simulink model "Demo_DSRC_BSM_Message_cs"  (Simulink 8.7)
settings: Solver=ode5  SolverMode=SingleTasking  StartTime=0.0  StopTime=10  FixedStep=1/20  RelTol=1e-3
PreLoadFcn:
  | check_NUTS_defined;
  | 
  | assignin('base',['model_closed_' bdroot],false);
InitFcn:
  | PreScanExperimentInitFcn(bdroot)
StopFcn:
  | PreScanExperimentStopFcn(bdroot)
undefined symbols (not defined in the file): spare_1, spare_10, spare_11, spare_12, spare_13, spare_14, spare_15, spare_16, spare_17, spare_18, spare_19, spare_2, spare_3, spare_4, spare_5, spare_6, spare_7, spare_8, spare_9
libraries: PreScanSimulinkLibrary x12, PreScanUsefulBlocks x4, simulink x2
(part 2 of 3)

== system Demo_DSRC_BSM_Message_cs/BMW_Z3_1/Trajectories ==
  Traj2State1 : Subsystem  Tag=Traj2State  mask(PreScan Demux Block:){}
      settings: DeleteFcn=PreScanBlockDeleteFcn;
  Trajectory_1 : Subsystem  Tag=Trajectory  mask(PreScan Source Block: Trajectory){FileName='Trajectory_1.mat', TimeStep=1/20}
      mask prompts: TimeStep "Time Step [s]"
      mask help:
      | The Trajectory block contains the trajectories defined in the PreScan Experiment Editor. The output of the trajectory block is the (vehicle) State.
      |
      | For more information, please click Help.
      mask init:
      | [direc,name]=fileparts(get_param(bdroot, 'FileName'));
      | load([direc,'/Trajectories/',FileName])
      | trajectory=trajectory';
      | 
      | traj.time=trajectory(:,1);%[];
      | traj.signals.values=trajectory(:,2:19);
      | traj.dimensions=18;
      | traj.label='';
      | 
      | SampleTime=traj.time(2)-traj.time(1);
      settings: DeleteFcn=PreScanBlockDeleteFcn;
      mask Help: eval('openHelp(312)')
      mask Display: fprintf(FileName)
  Trajectory_1_Offset : Constant  Tag=TrajectoryOffset  Value="[0  0  0  0  0  0]"
  State : Outport  Tag=TrajOutport
  wires:
  Trajectory_1/1(trajectory) -> Traj2State1/1(Traj Org)
  Trajectory_1_Offset/1 -> Traj2State1/2(Offset)
  Traj2State1/1(state) -> State/1

== system Demo_DSRC_BSM_Message_cs/Citroen_C3_1/DSRC Transmitter ==
  Data : Inport
  Enable : EnablePort  PropagateVarSize=During execution
  DSRC_T_BusAssignment : BusAssignment  Tag=BusDSRCT  AssignedSignals=spare_1,spare_2,spare_3,spare_4,spare_5,spare_6,spare_7,spare_8,spare_9,spare_10,spare_11,spare_12,spare_13,spare_14,spare_15,spare_16,spare_17,spare_18,spare_19
  DSRC_T_Mux : Subsystem  Tag=MuxDSRCT  mask(PreScan Mux Block:){}
      settings: DeleteFcn=PreScanBlockDeleteFcn;
      mask Display:
      | port_label('input', 1, 'Warning signal ID')
      | port_label('input', 2, 'Maneuvre ID')
      | port_label('input', 3, 'Vehicle Type')
      | port_label('input', 4, 'Braking Capacity')
      | port_label('input', 5, 'Vehicle Size')
      | port_label('input', 6, 'spare')
  Demux : Demux  Outputs=19
  Ground_{4..8} (5 alike) : Ground
  DSRC_T : Outport  Tag=AntennaTOutport
  wires:
  Demux/19 -> DSRC_T_BusAssignment/20  "Vehicle Height"
  Demux/18 -> DSRC_T_BusAssignment/19  "Vehicle Width"
  Demux/17 -> DSRC_T_BusAssignment/18  "Brakes"
  Demux/16 -> DSRC_T_BusAssignment/17  "Yaw rate"
  Demux/15 -> DSRC_T_BusAssignment/16  "Veritical Acc"
  Demux/14 -> DSRC_T_BusAssignment/15  "Lateral Acc"
  Demux/13 -> DSRC_T_BusAssignment/14  "Longitudinal Acc"
  Demux/12 -> DSRC_T_BusAssignment/13  "Angle"
  Demux/11 -> DSRC_T_BusAssignment/12  "Heading"
  Demux/10 -> DSRC_T_BusAssignment/11  "Speed"
  Demux/9 -> DSRC_T_BusAssignment/10  "Transmission State"
  Demux/8 -> DSRC_T_BusAssignment/9  "Accuracy"
  Demux/7 -> DSRC_T_BusAssignment/8  "Elevation"
  Demux/6 -> DSRC_T_BusAssignment/7  "Longitudinal"
  Demux/5 -> DSRC_T_BusAssignment/6  "Lateral"
  Ground_8/1 -> DSRC_T_Mux/5(vehicle_size)  "l50"
  Ground_7/1 -> DSRC_T_Mux/4(brakingcapacity)  "l49"
  Ground_6/1 -> DSRC_T_Mux/3(vehicle_type)  "l48"
  Ground_5/1 -> DSRC_T_Mux/2(maneuvre_id)  "l47"
  Ground_4/1 -> DSRC_T_Mux/1(warning_signal_id)  "l46"
  DSRC_T_Mux/1(Out1) -> DSRC_T/1  "l60"
  DSRC_T_BusAssignment/1 -> DSRC_T_Mux/6(spare)  "l58"
  Demux/4 -> DSRC_T_BusAssignment/5  "SecMark"
  Demux/3 -> DSRC_T_BusAssignment/4  "TempId"
  Demux/2 -> DSRC_T_BusAssignment/3  "MsgCount"
  Demux/1 -> DSRC_T_BusAssignment/2  "MsgId"
  Data/1 -> Demux/1
  DSRC_T_Mux/2(Out2) -> DSRC_T_BusAssignment/1  "L29"

== system Demo_DSRC_BSM_Message_cs/Citroen_C3_1/J2735 Encoder Basic Safety Message ==
  Msg : Inport
  Enable : EnablePort  PropagateVarSize=During execution
  Constant : Constant
  Demux : Demux  Outputs=19
  Embedded MATLAB Function : MATLAB Function  TreatAsAtomicUnit=on
  f() : Outport  InitialOutput=[1]
  Data : Outport  Port=2
  wires:
  Embedded MATLAB Function/1(y) -> Data/1
  Demux/19 -> Embedded MATLAB Function/19(u19)
  Demux/18 -> Embedded MATLAB Function/18(u18)
  Demux/17 -> Embedded MATLAB Function/17(u17)
  Demux/16 -> Embedded MATLAB Function/16(u16)
  Demux/15 -> Embedded MATLAB Function/15(u15)
  Demux/14 -> Embedded MATLAB Function/14(u14)
  Demux/13 -> Embedded MATLAB Function/13(u13)
  Demux/12 -> Embedded MATLAB Function/12(u12)
  Demux/11 -> Embedded MATLAB Function/11(u11)
  Demux/10 -> Embedded MATLAB Function/10(u10)
  Demux/9 -> Embedded MATLAB Function/9(u9)
  Demux/8 -> Embedded MATLAB Function/8(u8)
  Demux/7 -> Embedded MATLAB Function/7(u7)
  Demux/6 -> Embedded MATLAB Function/6(u6)
  Demux/5 -> Embedded MATLAB Function/5(u5)
  Demux/4 -> Embedded MATLAB Function/4(u4)
  Demux/3 -> Embedded MATLAB Function/3(u3)
  Demux/2 -> Embedded MATLAB Function/2(u2)
  Demux/1 -> Embedded MATLAB Function/1(u1)
  Constant/1 -> f()/1  "Enabled"
  Msg/1 -> Demux/1

== system Demo_DSRC_BSM_Message_cs/Citroen_C3_1/SELF_Demux ==
  SELF : Inport
  Demux1 : Demux  Outputs=3
  Demux2 : Demux  Outputs=3
  Demux3 : Demux  Outputs=[3 3 1 1]
  Demux4 : Demux  Outputs=3
  Gain : Gain  Gain=180/pi
  Gain1 : Gain  Gain=180/pi
  Selector : Selector  InputPortWidth=3  IndexOptions=Index vector (dialog)  Indices=[3]  OutputSizes=1
  compas converter : Subsystem
  xyz2GPS : PreScanUsefulBlocks/xyz2GPS  CoordinateCount=1  GPS_base=[0.000000 0.000000 0.000]
  x [m] : Outport
  y [m] : Outport  Port=2
  z [m] : Outport  Port=3
  rotx [deg] : Outport  Port=4
  roty [deg] : Outport  Port=5
  rotz [deg] : Outport  Port=6
  GPS lat [deg] : Outport  Port=7
  GPS long [deg] : Outport  Port=8
  GPS alt [m] : Outport  Port=9
  velocity [m/s] : Outport  Port=10
  heading [deg] : Outport  Port=11
  yaw rate [deg/s] : Outport  Port=12
  wires:
  Demux3/4 -> Gain1/1
  Gain1/1 -> yaw rate [deg/s]/1
  Demux3/3 -> velocity [m/s]/1
  compas converter/1(heading [deg]) -> heading [deg]/1
  xyz2GPS/1 -> Demux4/1
  Demux4/3 -> GPS alt [m]/1
  Demux4/2 -> GPS long [deg]/1
  Demux4/1 -> GPS lat [deg]/1
  Demux3/2 -> Gain/1, Selector/1
  Demux3/1 -> xyz2GPS/1, Demux1/1
  SELF/1 -> Demux3/1
  Demux2/3 -> rotz [deg]/1
  Demux2/2 -> roty [deg]/1
  Demux2/1 -> rotx [deg]/1
  Demux1/3 -> z [m]/1
  Demux1/2 -> y [m]/1
  Demux1/1 -> x [m]/1
  Gain/1 -> Demux2/1
  Selector/1 -> compas converter/1(rotz [rad])

== system Demo_DSRC_BSM_Message_cs/Citroen_C3_1/Trajectories ==
  Traj2State1 : Subsystem  Tag=Traj2State  mask(PreScan Demux Block:){}
      settings: DeleteFcn=PreScanBlockDeleteFcn;
  Trajectory_3 : Subsystem  Tag=Trajectory  mask(PreScan Source Block: Trajectory){FileName='Trajectory_3.mat', TimeStep=1/20}
      mask prompts: TimeStep "Time Step [s]"
      mask help:
      | The Trajectory block contains the trajectories defined in the PreScan Experiment Editor. The output of the trajectory block is the (vehicle) State.
      |
      | For more information, please click Help.
      mask init: same as Demo_DSRC_BSM_Message_cs/BMW_Z3_1/Trajectories/Trajectory_1
      settings: DeleteFcn=PreScanBlockDeleteFcn;
      mask Help: eval('openHelp(312)')
      mask Display: fprintf(FileName)
  Trajectory_3_Offset : Constant  Tag=TrajectoryOffset  Value="[0  0  0  0  0  0]"
  State : Outport  Tag=TrajOutport
  wires:
  Trajectory_3/1(trajectory) -> Traj2State1/1(Traj Org)
  Trajectory_3_Offset/1 -> Traj2State1/2(Offset)
  Traj2State1/1(state) -> State/1

== system Demo_DSRC_BSM_Message_cs/Fiat_Bravo_1/DSRC Transmitter ==
  Data : Inport
  Enable : EnablePort  PropagateVarSize=During execution
  DSRC_T_BusAssignment : BusAssignment  Tag=BusDSRCT  AssignedSignals=spare_1,spare_2,spare_3,spare_4,spare_5,spare_6,spare_7,spare_8,spare_9,spare_10,spare_11,spare_12,spare_13,spare_14,spare_15,spare_16,spare_17,spare_18,spare_19
  DSRC_T_Mux : Subsystem  Tag=MuxDSRCT  mask(PreScan Mux Block:){}
      settings: DeleteFcn=PreScanBlockDeleteFcn;
      mask Display:
      | port_label('input', 1, 'Warning signal ID')
      | port_label('input', 2, 'Maneuvre ID')
      | port_label('input', 3, 'Vehicle Type')
      | port_label('input', 4, 'Braking Capacity')
      | port_label('input', 5, 'Vehicle Size')
      | port_label('input', 6, 'spare')
  Demux : Demux  Outputs=19
  Ground_{4..8} (5 alike) : Ground
  DSRC_T : Outport  Tag=AntennaTOutport
  wires:
  Demux/19 -> DSRC_T_BusAssignment/20  "Vehicle Height"
  Demux/18 -> DSRC_T_BusAssignment/19  "Vehicle Width"
  Demux/17 -> DSRC_T_BusAssignment/18  "Brakes"
  Demux/16 -> DSRC_T_BusAssignment/17  "Yaw rate"
  Demux/15 -> DSRC_T_BusAssignment/16  "Veritical Acc"
  Demux/14 -> DSRC_T_BusAssignment/15  "Lateral Acc"
  Demux/13 -> DSRC_T_BusAssignment/14  "Longitudinal Acc"
  Demux/12 -> DSRC_T_BusAssignment/13  "Angle"
  Demux/11 -> DSRC_T_BusAssignment/12  "Heading"
  Demux/10 -> DSRC_T_BusAssignment/11  "Speed"
  Demux/9 -> DSRC_T_BusAssignment/10  "Transmission State"
  Demux/8 -> DSRC_T_BusAssignment/9  "Accuracy"
  Demux/7 -> DSRC_T_BusAssignment/8  "Elevation"
  Demux/6 -> DSRC_T_BusAssignment/7  "Longitudinal"
  Demux/5 -> DSRC_T_BusAssignment/6  "Lateral"
  Ground_8/1 -> DSRC_T_Mux/5(vehicle_size)  "l50"
  Ground_7/1 -> DSRC_T_Mux/4(brakingcapacity)  "l49"
  Ground_6/1 -> DSRC_T_Mux/3(vehicle_type)  "l48"
  Ground_5/1 -> DSRC_T_Mux/2(maneuvre_id)  "l47"
  Ground_4/1 -> DSRC_T_Mux/1(warning_signal_id)  "l46"
  DSRC_T_Mux/1(Out1) -> DSRC_T/1  "l60"
  DSRC_T_BusAssignment/1 -> DSRC_T_Mux/6(spare)  "l58"
  Demux/4 -> DSRC_T_BusAssignment/5  "SecMark"
  Demux/3 -> DSRC_T_BusAssignment/4  "TempId"
  Demux/2 -> DSRC_T_BusAssignment/3  "MsgCount"
  Demux/1 -> DSRC_T_BusAssignment/2  "MsgId"
  Data/1 -> Demux/1
  DSRC_T_Mux/2(Out2) -> DSRC_T_BusAssignment/1  "L29"

== system Demo_DSRC_BSM_Message_cs/Fiat_Bravo_1/J2735 Encoder Basic Safety Message ==
  Msg : Inport
  Enable : EnablePort  PropagateVarSize=During execution
  Constant : Constant
  Demux : Demux  Outputs=19
  Embedded MATLAB Function : MATLAB Function  TreatAsAtomicUnit=on
  f() : Outport  InitialOutput=[1]
  Data : Outport  Port=2
  wires:
  Embedded MATLAB Function/1(y) -> Data/1
  Demux/19 -> Embedded MATLAB Function/19(u19)
  Demux/18 -> Embedded MATLAB Function/18(u18)
  Demux/17 -> Embedded MATLAB Function/17(u17)
  Demux/16 -> Embedded MATLAB Function/16(u16)
  Demux/15 -> Embedded MATLAB Function/15(u15)
  Demux/14 -> Embedded MATLAB Function/14(u14)
  Demux/13 -> Embedded MATLAB Function/13(u13)
  Demux/12 -> Embedded MATLAB Function/12(u12)
  Demux/11 -> Embedded MATLAB Function/11(u11)
  Demux/10 -> Embedded MATLAB Function/10(u10)
  Demux/9 -> Embedded MATLAB Function/9(u9)
  Demux/8 -> Embedded MATLAB Function/8(u8)
  Demux/7 -> Embedded MATLAB Function/7(u7)
  Demux/6 -> Embedded MATLAB Function/6(u6)
  Demux/5 -> Embedded MATLAB Function/5(u5)
  Demux/4 -> Embedded MATLAB Function/4(u4)
  Demux/3 -> Embedded MATLAB Function/3(u3)
  Demux/2 -> Embedded MATLAB Function/2(u2)
  Demux/1 -> Embedded MATLAB Function/1(u1)
  Constant/1 -> f()/1  "Enabled"
  Msg/1 -> Demux/1

== system Demo_DSRC_BSM_Message_cs/Fiat_Bravo_1/SELF_Demux ==
  SELF : Inport
  Demux1 : Demux  Outputs=3
  Demux2 : Demux  Outputs=3
  Demux3 : Demux  Outputs=[3 3 1 1]
  Demux4 : Demux  Outputs=3
  Gain : Gain  Gain=180/pi
  Gain1 : Gain  Gain=180/pi
  Selector : Selector  InputPortWidth=3  IndexOptions=Index vector (dialog)  Indices=[3]  OutputSizes=1
  compas converter : Subsystem
  xyz2GPS : PreScanUsefulBlocks/xyz2GPS  CoordinateCount=1  GPS_base=[0.000000 0.000000 0.000]
  x [m] : Outport
  y [m] : Outport  Port=2
  z [m] : Outport  Port=3
  rotx [deg] : Outport  Port=4
  roty [deg] : Outport  Port=5
  rotz [deg] : Outport  Port=6
  GPS lat [deg] : Outport  Port=7
  GPS long [deg] : Outport  Port=8
  GPS alt [m] : Outport  Port=9
  velocity [m/s] : Outport  Port=10
  heading [deg] : Outport  Port=11
  yaw rate [deg/s] : Outport  Port=12
  wires:
  Demux3/4 -> Gain1/1
  Gain1/1 -> yaw rate [deg/s]/1
  Demux3/3 -> velocity [m/s]/1
  compas converter/1(heading [deg]) -> heading [deg]/1
  xyz2GPS/1 -> Demux4/1
  Demux4/3 -> GPS alt [m]/1
  Demux4/2 -> GPS long [deg]/1
  Demux4/1 -> GPS lat [deg]/1
  Demux3/2 -> Gain/1, Selector/1
  Demux3/1 -> xyz2GPS/1, Demux1/1
  SELF/1 -> Demux3/1
  Demux2/3 -> rotz [deg]/1
  Demux2/2 -> roty [deg]/1
  Demux2/1 -> rotx [deg]/1
  Demux1/3 -> z [m]/1
  Demux1/2 -> y [m]/1
  Demux1/1 -> x [m]/1
  Gain/1 -> Demux2/1
  Selector/1 -> compas converter/1(rotz [rad])

== system Demo_DSRC_BSM_Message_cs/Fiat_Bravo_1/Trajectories ==
  Traj2State1 : Subsystem  Tag=Traj2State  mask(PreScan Demux Block:){}
      settings: DeleteFcn=PreScanBlockDeleteFcn;
  Trajectory_2 : Subsystem  Tag=Trajectory  mask(PreScan Source Block: Trajectory){FileName='Trajectory_2.mat', TimeStep=1/20}
      mask prompts: TimeStep "Time Step [s]"
      mask help:
      | The Trajectory block contains the trajectories defined in the PreScan Experiment Editor. The output of the trajectory block is the (vehicle) State.
      |
      | For more information, please click Help.
      mask init: same as Demo_DSRC_BSM_Message_cs/BMW_Z3_1/Trajectories/Trajectory_1
      settings: DeleteFcn=PreScanBlockDeleteFcn;
      mask Help: eval('openHelp(312)')
      mask Display: fprintf(FileName)
  Trajectory_2_Offset : Constant  Tag=TrajectoryOffset  Value="[0  0  0  0  0  0]"
  State : Outport  Tag=TrajOutport
  wires:
  Trajectory_2/1(trajectory) -> Traj2State1/1(Traj Org)
  Trajectory_2_Offset/1 -> Traj2State1/2(Offset)
  Traj2State1/1(state) -> State/1

== system Demo_DSRC_BSM_Message_cs/STATE_BMW_Z3_1/Acceleration ==
  Y : Inport
  Assignment : Assignment  IndexMode=Zero-based  SampleTime=TimeStep  IndexOptions=Starting index (dialog)  Indices=PortIndex  OutputSizes=[1 1]
  Data Store Read : DataStoreRead  DataStoreName=SimCoreActuators  SampleTime=TimeStep
  Data Store Write : DataStoreWrite  DataStoreName=SimCoreActuators
  wires:
  Assignment/1 -> Data Store Write/1
  Data Store Read/1 -> Assignment/1
  Y/1 -> Assignment/2

== system Demo_DSRC_BSM_Message_cs/STATE_BMW_Z3_1/Position ==
  Y : Inport
  Assignment : Assignment  IndexMode=Zero-based  SampleTime=TimeStep  IndexOptions=Starting index (dialog)  Indices=PortIndex  OutputSizes=[1 1]
  Data Store Read : DataStoreRead  DataStoreName=SimCoreActuators  SampleTime=TimeStep
  Data Store Write : DataStoreWrite  DataStoreName=SimCoreActuators
  wires:
  Y/1 -> Assignment/2
  Data Store Read/1 -> Assignment/1
  Assignment/1 -> Data Store Write/1

== system Demo_DSRC_BSM_Message_cs/STATE_BMW_Z3_1/RPY ==
  Y : Inport
  Assignment : Assignment  IndexMode=Zero-based  SampleTime=TimeStep  IndexOptions=Starting index (dialog)  Indices=PortIndex  OutputSizes=[1 1]
  Data Store Read : DataStoreRead  DataStoreName=SimCoreActuators  SampleTime=TimeStep
  Data Store Write : DataStoreWrite  DataStoreName=SimCoreActuators
  wires:
  Assignment/1 -> Data Store Write/1
  Data Store Read/1 -> Assignment/1
  Y/1 -> Assignment/2

== system Demo_DSRC_BSM_Message_cs/STATE_BMW_Z3_1/Velocity ==
  Y : Inport
  Assignment : Assignment  IndexMode=Zero-based  SampleTime=TimeStep  IndexOptions=Starting index (dialog)  Indices=PortIndex  OutputSizes=[1 1]
  Data Store Read : DataStoreRead  DataStoreName=SimCoreActuators  SampleTime=TimeStep
  Data Store Write : DataStoreWrite  DataStoreName=SimCoreActuators
  wires:
  Assignment/1 -> Data Store Write/1
  Data Store Read/1 -> Assignment/1
  Y/1 -> Assignment/2

== system Demo_DSRC_BSM_Message_cs/STATE_BMW_Z3_1/velRPY ==
  Y : Inport
  Assignment : Assignment  IndexMode=Zero-based  SampleTime=TimeStep  IndexOptions=Starting index (dialog)  Indices=PortIndex  OutputSizes=[1 1]
  Data Store Read : DataStoreRead  DataStoreName=SimCoreActuators  SampleTime=TimeStep
  Data Store Write : DataStoreWrite  DataStoreName=SimCoreActuators
  wires:
  Assignment/1 -> Data Store Write/1
  Data Store Read/1 -> Assignment/1
  Y/1 -> Assignment/2

== system Demo_DSRC_BSM_Message_cs/STATE_Citroen_C3_1/Acceleration ==
  Y : Inport
  Assignment : Assignment  IndexMode=Zero-based  SampleTime=TimeStep  IndexOptions=Starting index (dialog)  Indices=PortIndex  OutputSizes=[1 1]
  Data Store Read : DataStoreRead  DataStoreName=SimCoreActuators  SampleTime=TimeStep
  Data Store Write : DataStoreWrite  DataStoreName=SimCoreActuators
  wires:
  Assignment/1 -> Data Store Write/1
  Data Store Read/1 -> Assignment/1
  Y/1 -> Assignment/2

== system Demo_DSRC_BSM_Message_cs/STATE_Citroen_C3_1/Position ==
  Y : Inport
  Assignment : Assignment  IndexMode=Zero-based  SampleTime=TimeStep  IndexOptions=Starting index (dialog)  Indices=PortIndex  OutputSizes=[1 1]
  Data Store Read : DataStoreRead  DataStoreName=SimCoreActuators  SampleTime=TimeStep
  Data Store Write : DataStoreWrite  DataStoreName=SimCoreActuators
  wires:
  Y/1 -> Assignment/2
  Data Store Read/1 -> Assignment/1
  Assignment/1 -> Data Store Write/1

== system Demo_DSRC_BSM_Message_cs/STATE_Citroen_C3_1/RPY ==
  Y : Inport
  Assignment : Assignment  IndexMode=Zero-based  SampleTime=TimeStep  IndexOptions=Starting index (dialog)  Indices=PortIndex  OutputSizes=[1 1]
  Data Store Read : DataStoreRead  DataStoreName=SimCoreActuators  SampleTime=TimeStep
  Data Store Write : DataStoreWrite  DataStoreName=SimCoreActuators
  wires:
  Assignment/1 -> Data Store Write/1
  Data Store Read/1 -> Assignment/1
  Y/1 -> Assignment/2

== system Demo_DSRC_BSM_Message_cs/STATE_Citroen_C3_1/Velocity ==
  Y : Inport
  Assignment : Assignment  IndexMode=Zero-based  SampleTime=TimeStep  IndexOptions=Starting index (dialog)  Indices=PortIndex  OutputSizes=[1 1]
  Data Store Read : DataStoreRead  DataStoreName=SimCoreActuators  SampleTime=TimeStep
  Data Store Write : DataStoreWrite  DataStoreName=SimCoreActuators
  wires:
  Assignment/1 -> Data Store Write/1
  Data Store Read/1 -> Assignment/1
  Y/1 -> Assignment/2

== system Demo_DSRC_BSM_Message_cs/STATE_Citroen_C3_1/velRPY ==
  Y : Inport
  Assignment : Assignment  IndexMode=Zero-based  SampleTime=TimeStep  IndexOptions=Starting index (dialog)  Indices=PortIndex  OutputSizes=[1 1]
  Data Store Read : DataStoreRead  DataStoreName=SimCoreActuators  SampleTime=TimeStep
  Data Store Write : DataStoreWrite  DataStoreName=SimCoreActuators
  wires:
  Assignment/1 -> Data Store Write/1
  Data Store Read/1 -> Assignment/1
  Y/1 -> Assignment/2

== system Demo_DSRC_BSM_Message_cs/STATE_Fiat_Bravo_1/Acceleration ==
  Y : Inport
  Assignment : Assignment  IndexMode=Zero-based  SampleTime=TimeStep  IndexOptions=Starting index (dialog)  Indices=PortIndex  OutputSizes=[1 1]
  Data Store Read : DataStoreRead  DataStoreName=SimCoreActuators  SampleTime=TimeStep
  Data Store Write : DataStoreWrite  DataStoreName=SimCoreActuators
  wires:
  Assignment/1 -> Data Store Write/1
  Data Store Read/1 -> Assignment/1
  Y/1 -> Assignment/2

== system Demo_DSRC_BSM_Message_cs/STATE_Fiat_Bravo_1/Position ==
  Y : Inport
  Assignment : Assignment  IndexMode=Zero-based  SampleTime=TimeStep  IndexOptions=Starting index (dialog)  Indices=PortIndex  OutputSizes=[1 1]
  Data Store Read : DataStoreRead  DataStoreName=SimCoreActuators  SampleTime=TimeStep
  Data Store Write : DataStoreWrite  DataStoreName=SimCoreActuators
  wires:
  Y/1 -> Assignment/2
  Data Store Read/1 -> Assignment/1
  Assignment/1 -> Data Store Write/1

== system Demo_DSRC_BSM_Message_cs/STATE_Fiat_Bravo_1/RPY ==
  Y : Inport
  Assignment : Assignment  IndexMode=Zero-based  SampleTime=TimeStep  IndexOptions=Starting index (dialog)  Indices=PortIndex  OutputSizes=[1 1]
  Data Store Read : DataStoreRead  DataStoreName=SimCoreActuators  SampleTime=TimeStep
  Data Store Write : DataStoreWrite  DataStoreName=SimCoreActuators
  wires:
  Assignment/1 -> Data Store Write/1
  Data Store Read/1 -> Assignment/1
  Y/1 -> Assignment/2

== system Demo_DSRC_BSM_Message_cs/STATE_Fiat_Bravo_1/Velocity ==
  Y : Inport
  Assignment : Assignment  IndexMode=Zero-based  SampleTime=TimeStep  IndexOptions=Starting index (dialog)  Indices=PortIndex  OutputSizes=[1 1]
  Data Store Read : DataStoreRead  DataStoreName=SimCoreActuators  SampleTime=TimeStep
  Data Store Write : DataStoreWrite  DataStoreName=SimCoreActuators
  wires:
  Assignment/1 -> Data Store Write/1
  Data Store Read/1 -> Assignment/1
  Y/1 -> Assignment/2

== system Demo_DSRC_BSM_Message_cs/STATE_Fiat_Bravo_1/velRPY ==
  Y : Inport
  Assignment : Assignment  IndexMode=Zero-based  SampleTime=TimeStep  IndexOptions=Starting index (dialog)  Indices=PortIndex  OutputSizes=[1 1]
  Data Store Read : DataStoreRead  DataStoreName=SimCoreActuators  SampleTime=TimeStep
  Data Store Write : DataStoreWrite  DataStoreName=SimCoreActuators
  wires:
  Assignment/1 -> Data Store Write/1
  Data Store Read/1 -> Assignment/1
  Y/1 -> Assignment/2

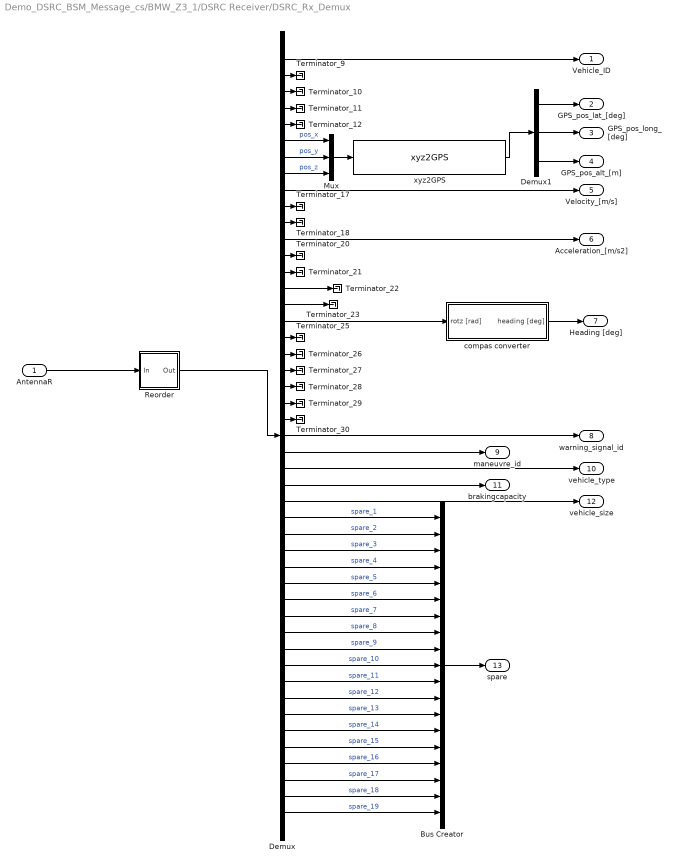
== system Demo_DSRC_BSM_Message_cs/BMW_Z3_1/DSRC Receiver/DSRC_Rx_Demux ==
  AntennaR : Inport
  Bus Creator : BusCreator  Inputs=19
  Demux : Demux  Outputs=47
  Demux1 : Demux  Outputs=3
  Mux : Mux  Inputs=3
  Reorder : Subsystem  mask(Output reorder block){NrOfOutputs=47, NrOfObjects=2}
      mask prompts: NrOfOutputs "Number Of Outputs [-]"; NrOfObjects "Number Of Objects [-]"
      mask help: Change output order from object based to output type based
      mask init:
      | InputPortWidth=NrOfObjects*NrOfOutputs;
      | Input=1:InputPortWidth;
      | ReshapedInput=reshape(Input,NrOfOutputs,NrOfObjects);
      | TransposedReshapedInput=transpose(ReshapedInput);
      | Elements=reshape(TransposedReshapedInput,length(Input),1);
  Terminator_{9..12,17..18,20..23,25..30} (16 alike) : Terminator
  compas converter : Subsystem
  xyz2GPS : PreScanUsefulBlocks/xyz2GPS  CoordinateCount=2  GPS_base=[0.000000 0.000000 0.000]
  Vehicle_ID : Outport
  GPS_pos_lat_[deg] : Outport  Port=2
  GPS_pos_long_[deg] : Outport  Port=3
  GPS_pos_alt_[m] : Outport  Port=4
  Velocity_[m/s] : Outport  Port=5
  Acceleration_[m/s2] : Outport  Port=6
  Heading [deg] : Outport  Port=7
  warning_signal_id : Outport  Port=8
  maneuvre_id : Outport  Port=9
  vehicle_type : Outport  Port=10
  brakingcapacity : Outport  Port=11
  vehicle_size : Outport  Port=12
  spare : Outport  Port=13
  wires:
  Demux/47 -> Bus Creator/19  "spare_19"
  Demux/46 -> Bus Creator/18  "spare_18"
  Demux/45 -> Bus Creator/17  "spare_17"
  Demux/44 -> Bus Creator/16  "spare_16"
  Demux/43 -> Bus Creator/15  "spare_15"
  Demux/42 -> Bus Creator/14  "spare_14"
  Demux/41 -> Bus Creator/13  "spare_13"
  Demux/40 -> Bus Creator/12  "spare_12"
  Demux/39 -> Bus Creator/11  "spare_11"
  Demux/38 -> Bus Creator/10  "spare_10"
  Demux/37 -> Bus Creator/9  "spare_9"
  Demux/36 -> Bus Creator/8  "spare_8"
  Demux/35 -> Bus Creator/7  "spare_7"
  Demux/34 -> Bus Creator/6  "spare_6"
  Demux/33 -> Bus Creator/5  "spare_5"
  Demux/32 -> Bus Creator/4  "spare_4"
  Demux/31 -> Bus Creator/3  "spare_3"
  Demux/30 -> Bus Creator/2  "spare_2"
  Demux/29 -> Bus Creator/1  "spare_1"
  AntennaR/1 -> Reorder/1(In)
  Reorder/1(Out) -> Demux/1
  Mux/1 -> xyz2GPS/1
  Demux1/3 -> GPS_pos_alt_[m]/1
  Demux1/2 -> GPS_pos_long_[deg]/1
  Demux1/1 -> GPS_pos_lat_[deg]/1
  xyz2GPS/1 -> Demux1/1
  Demux/28 -> vehicle_size/1
  Demux/27 -> brakingcapacity/1
  Demux/26 -> vehicle_type/1
  Demux/25 -> maneuvre_id/1
  Demux/24 -> warning_signal_id/1
  Demux/9 -> Velocity_[m/s]/1
  Demux/23 -> Terminator_30/1
  Demux/22 -> Terminator_29/1
  Demux/21 -> Terminator_28/1
  Demux/20 -> Terminator_27/1
  Demux/19 -> Terminator_26/1
  Demux/18 -> Terminator_25/1
  Demux/17 -> compas converter/1(rotz [rad])
  Demux/16 -> Terminator_23/1
  Demux/15 -> Terminator_22/1
  Demux/14 -> Terminator_21/1
  Demux/13 -> Terminator_20/1
  Demux/12 -> Acceleration_[m/s2]/1
  Demux/11 -> Terminator_18/1
  Demux/10 -> Terminator_17/1
  Demux/8 -> Mux/3  "pos_z"
  Demux/7 -> Mux/2  "pos_y"
  Demux/6 -> Mux/1  "pos_x"
  Demux/5 -> Terminator_12/1
  Demux/4 -> Terminator_11/1
  Demux/3 -> Terminator_10/1
  Demux/2 -> Terminator_9/1
  Demux/1 -> Vehicle_ID/1
  compas converter/1(heading [deg]) -> Heading [deg]/1
  Bus Creator/1 -> spare/1

== system Demo_DSRC_BSM_Message_cs/BMW_Z3_1/SELF_Demux/compas converter ==
  rotz [rad] : Inport
  cart2compas : Subsystem
  rad2deg : Gain  Gain=180/pi
  heading [deg] : Outport
  wires:
  cart2compas/1(heading [deg]) -> heading [deg]/1
  rotz [rad]/1 -> rad2deg/1
  rad2deg/1 -> cart2compas/1(Angle [deg])

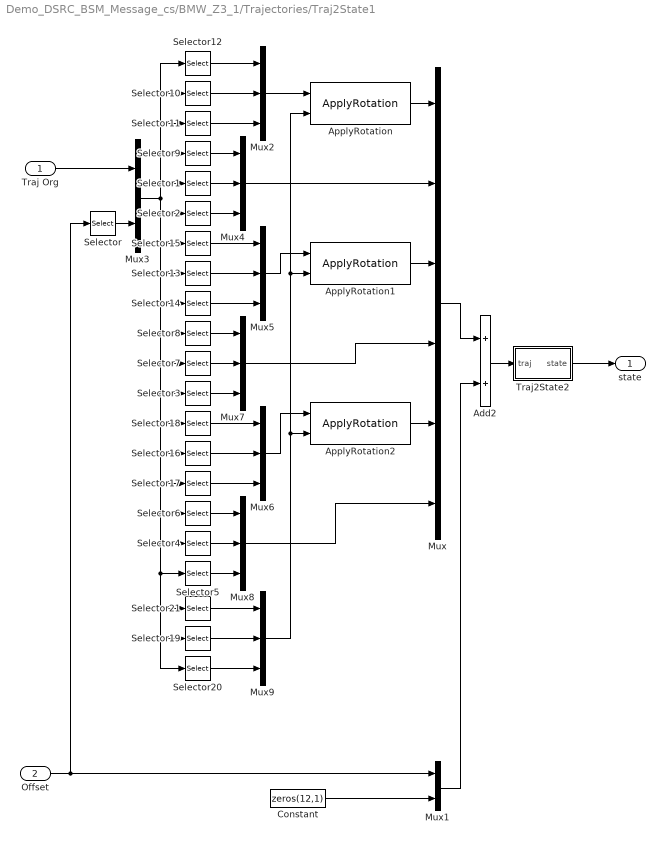
== system Demo_DSRC_BSM_Message_cs/BMW_Z3_1/Trajectories/Traj2State1 ==
  Traj Org : Inport
  Offset : Inport  Port=2
  Add2 : Sum
  ApplyRotation : PreScanSimulinkLibrary/ApplyRotation
  ApplyRotation1 : PreScanSimulinkLibrary/ApplyRotation
  ApplyRotation2 : PreScanSimulinkLibrary/ApplyRotation
  Constant : Constant  Value=zeros(12,1)
  Mux : Mux  Inputs=6
  Mux1 : Mux  Inputs=2
  Mux{2,4..9} (7 alike) : Mux  Inputs=3
  Mux3 : Mux  Inputs=2
  Selector : Selector  InputPortWidth=6  IndexOptions=Index vector (dialog)  Indices=[4 5 6]  OutputSizes=1
  Selector1 : Selector  InputPortWidth=21  IndexOptions=Index vector (dialog)  Indices=[5]  OutputSizes=1
  Selector10 : Selector  InputPortWidth=21  IndexOptions=Index vector (dialog)  Indices=[2]  OutputSizes=1
  Selector11 : Selector  InputPortWidth=21  IndexOptions=Index vector (dialog)  Indices=[3]  OutputSizes=1
  Selector12 : Selector  InputPortWidth=21  IndexOptions=Index vector (dialog)  Indices=[1]  OutputSizes=1
  Selector13 : Selector  InputPortWidth=21  IndexOptions=Index vector (dialog)  Indices=[8]  OutputSizes=1
  Selector14 : Selector  InputPortWidth=21  IndexOptions=Index vector (dialog)  Indices=[9]  OutputSizes=1
  Selector15 : Selector  InputPortWidth=21  IndexOptions=Index vector (dialog)  Indices=[7]  OutputSizes=1
  Selector16 : Selector  InputPortWidth=21  IndexOptions=Index vector (dialog)  Indices=[14]  OutputSizes=1
  Selector17 : Selector  InputPortWidth=21  IndexOptions=Index vector (dialog)  Indices=[15]  OutputSizes=1
  Selector18 : Selector  InputPortWidth=21  IndexOptions=Index vector (dialog)  Indices=[13]  OutputSizes=1
  Selector19 : Selector  InputPortWidth=21  IndexOptions=Index vector (dialog)  Indices=[20]  OutputSizes=1
  Selector2 : Selector  InputPortWidth=21  IndexOptions=Index vector (dialog)  Indices=[6]  OutputSizes=1
  Selector20 : Selector  InputPortWidth=21  IndexOptions=Index vector (dialog)  Indices=[21]  OutputSizes=1
  Selector21 : Selector  InputPortWidth=21  IndexOptions=Index vector (dialog)  Indices=[19]  OutputSizes=1
  Selector3 : Selector  InputPortWidth=21  IndexOptions=Index vector (dialog)  Indices=[12]  OutputSizes=1
  Selector4 : Selector  InputPortWidth=21  IndexOptions=Index vector (dialog)  Indices=[17]  OutputSizes=1
  Selector5 : Selector  InputPortWidth=21  IndexOptions=Index vector (dialog)  Indices=[18]  OutputSizes=1
  Selector6 : Selector  InputPortWidth=21  IndexOptions=Index vector (dialog)  Indices=[16]  OutputSizes=1
  Selector7 : Selector  InputPortWidth=21  IndexOptions=Index vector (dialog)  Indices=[11]  OutputSizes=1
  Selector8 : Selector  InputPortWidth=21  IndexOptions=Index vector (dialog)  Indices=[10]  OutputSizes=1
  Selector9 : Selector  InputPortWidth=21  IndexOptions=Index vector (dialog)  Indices=[4]  OutputSizes=1
  Traj2State2 : Subsystem
  state : Outport
  wires:
  Mux9/1 -> ApplyRotation2/2, ApplyRotation1/2, ApplyRotation/2
  Selector20/1 -> Mux9/3
  Selector19/1 -> Mux9/2
  Selector21/1 -> Mux9/1
  Selector5/1 -> Mux8/3
  Selector4/1 -> Mux8/2
  Selector6/1 -> Mux8/1
  Mux8/1 -> Mux/6
  Mux6/1 -> ApplyRotation2/1
  Mux7/1 -> Mux/4
  ApplyRotation2/1 -> Mux/5
  Selector3/1 -> Mux7/3
  Selector7/1 -> Mux7/2
  Selector8/1 -> Mux7/1
  Mux4/1 -> Mux/2
  Mux5/1 -> ApplyRotation1/1
  ApplyRotation1/1 -> Mux/3
  Mux2/1 -> ApplyRotation/1
  ApplyRotation/1 -> Mux/1
  Selector2/1 -> Mux4/3
  Selector1/1 -> Mux4/2
  Selector9/1 -> Mux4/1
  Selector17/1 -> Mux6/3
  Selector16/1 -> Mux6/2
  Selector18/1 -> Mux6/1
  Selector14/1 -> Mux5/3
  Selector13/1 -> Mux5/2
  Selector15/1 -> Mux5/1
  Selector11/1 -> Mux2/3
  Selector10/1 -> Mux2/2
  Selector12/1 -> Mux2/1
  Mux3/1 -> Selector8/1, Selector7/1, Selector3/1, Selector18/1, Selector16/1, Selector17/1, Selector6/1, Selector20/1, Selector19/1, Selector21/1, Selector5/1, Selector4/1, Selector14/1, Selector13/1, Selector15/1, Selector2/1, Selector1/1, Selector9/1, Selector12/1, Selector10/1, Selector11/1
  Mux1/1 -> Add2/2
  Constant/1 -> Mux1/2
  Add2/1 -> Traj2State2/1(traj)
  Selector/1 -> Mux3/2
  Traj Org/1 -> Mux3/1
  Offset/1 -> Mux1/1, Selector/1
  Mux/1 -> Add2/1
  Traj2State2/1(state) -> state/1

== system Demo_DSRC_BSM_Message_cs/BMW_Z3_1/Trajectories/Trajectory_1 ==
  From Workspace : FromWorkspace  VariableName=trajectory  SampleTime=TimeStep  OutputAfterFinalValue=Holding final value
  From Workspace1 : FromWorkspace  VariableName=trajectory  SampleTime=TimeStep  OutputAfterFinalValue=Setting to zero
  Mux : Mux  Inputs=2
  Selector1 : Selector  InputPortWidth=24  IndexOptions=Index vector (dialog)  Indices=[7:18]  OutputSizes=1
  Selector9 : Selector  InputPortWidth=24  IndexOptions=Index vector (dialog)  Indices=[1:6]  OutputSizes=1
  trajectory : Outport
  wires:
  Selector1/1 -> Mux/2
  Selector9/1 -> Mux/1
  Mux/1 -> trajectory/1
  From Workspace1/1 -> Selector1/1
  From Workspace/1 -> Selector9/1

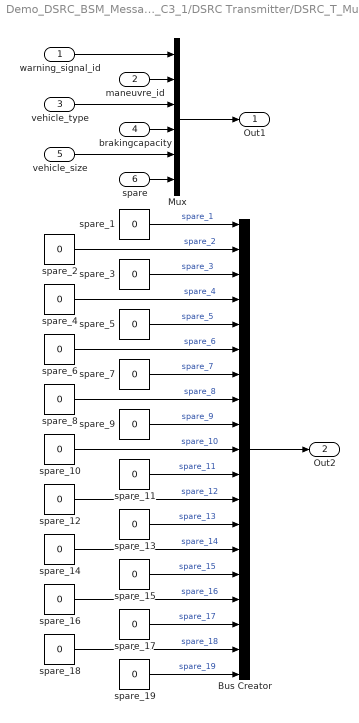
== system Demo_DSRC_BSM_Message_cs/Citroen_C3_1/DSRC Transmitter/DSRC_T_Mux ==
  warning_signal_id : Inport
  maneuvre_id : Inport  Port=2
  vehicle_type : Inport  Port=3
  brakingcapacity : Inport  Port=4
  vehicle_size : Inport  Port=5
  spare : Inport  Port=6
  Bus Creator : BusCreator  Inputs=19
  Mux : Mux  Inputs=6
  spare_{1..19} (19 alike) : Constant  Value=0
  Out1 : Outport
  Out2 : Outport  Port=2
  wires:
  spare_3/1 -> Bus Creator/3  "spare_3"
  spare_2/1 -> Bus Creator/2  "spare_2"
  spare_1/1 -> Bus Creator/1  "spare_1"
  spare_4/1 -> Bus Creator/4  "spare_4"
  spare/1 -> Mux/6
  Bus Creator/1 -> Out2/1
  Mux/1 -> Out1/1
  vehicle_size/1 -> Mux/5
  brakingcapacity/1 -> Mux/4
  vehicle_type/1 -> Mux/3
  maneuvre_id/1 -> Mux/2
  warning_signal_id/1 -> Mux/1
  spare_5/1 -> Bus Creator/5  "spare_5"
  spare_6/1 -> Bus Creator/6  "spare_6"
  spare_7/1 -> Bus Creator/7  "spare_7"
  spare_8/1 -> Bus Creator/8  "spare_8"
  spare_9/1 -> Bus Creator/9  "spare_9"
  spare_10/1 -> Bus Creator/10  "spare_10"
  spare_11/1 -> Bus Creator/11  "spare_11"
  spare_12/1 -> Bus Creator/12  "spare_12"
  spare_13/1 -> Bus Creator/13  "spare_13"
  spare_14/1 -> Bus Creator/14  "spare_14"
  spare_15/1 -> Bus Creator/15  "spare_15"
  spare_16/1 -> Bus Creator/16  "spare_16"
  spare_17/1 -> Bus Creator/17  "spare_17"
  spare_18/1 -> Bus Creator/18  "spare_18"
  spare_19/1 -> Bus Creator/19  "spare_19"

== system Demo_DSRC_BSM_Message_cs/Citroen_C3_1/SELF_Demux/compas converter ==
  rotz [rad] : Inport
  cart2compas : Subsystem
  rad2deg : Gain  Gain=180/pi
  heading [deg] : Outport
  wires:
  cart2compas/1(heading [deg]) -> heading [deg]/1
  rotz [rad]/1 -> rad2deg/1
  rad2deg/1 -> cart2compas/1(Angle [deg])

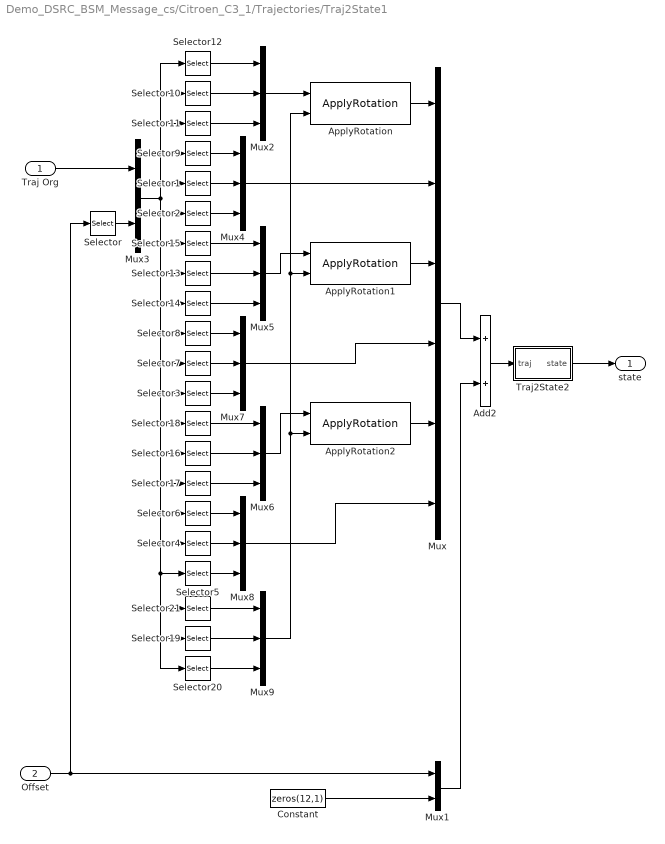
== system Demo_DSRC_BSM_Message_cs/Citroen_C3_1/Trajectories/Traj2State1 ==
  Traj Org : Inport
  Offset : Inport  Port=2
  Add2 : Sum
  ApplyRotation : PreScanSimulinkLibrary/ApplyRotation
  ApplyRotation1 : PreScanSimulinkLibrary/ApplyRotation
  ApplyRotation2 : PreScanSimulinkLibrary/ApplyRotation
  Constant : Constant  Value=zeros(12,1)
  Mux : Mux  Inputs=6
  Mux1 : Mux  Inputs=2
  Mux{2,4..9} (7 alike) : Mux  Inputs=3
  Mux3 : Mux  Inputs=2
  Selector : Selector  InputPortWidth=6  IndexOptions=Index vector (dialog)  Indices=[4 5 6]  OutputSizes=1
  Selector1 : Selector  InputPortWidth=21  IndexOptions=Index vector (dialog)  Indices=[5]  OutputSizes=1
  Selector10 : Selector  InputPortWidth=21  IndexOptions=Index vector (dialog)  Indices=[2]  OutputSizes=1
  Selector11 : Selector  InputPortWidth=21  IndexOptions=Index vector (dialog)  Indices=[3]  OutputSizes=1
  Selector12 : Selector  InputPortWidth=21  IndexOptions=Index vector (dialog)  Indices=[1]  OutputSizes=1
  Selector13 : Selector  InputPortWidth=21  IndexOptions=Index vector (dialog)  Indices=[8]  OutputSizes=1
  Selector14 : Selector  InputPortWidth=21  IndexOptions=Index vector (dialog)  Indices=[9]  OutputSizes=1
  Selector15 : Selector  InputPortWidth=21  IndexOptions=Index vector (dialog)  Indices=[7]  OutputSizes=1
  Selector16 : Selector  InputPortWidth=21  IndexOptions=Index vector (dialog)  Indices=[14]  OutputSizes=1
  Selector17 : Selector  InputPortWidth=21  IndexOptions=Index vector (dialog)  Indices=[15]  OutputSizes=1
  Selector18 : Selector  InputPortWidth=21  IndexOptions=Index vector (dialog)  Indices=[13]  OutputSizes=1
  Selector19 : Selector  InputPortWidth=21  IndexOptions=Index vector (dialog)  Indices=[20]  OutputSizes=1
  Selector2 : Selector  InputPortWidth=21  IndexOptions=Index vector (dialog)  Indices=[6]  OutputSizes=1
  Selector20 : Selector  InputPortWidth=21  IndexOptions=Index vector (dialog)  Indices=[21]  OutputSizes=1
  Selector21 : Selector  InputPortWidth=21  IndexOptions=Index vector (dialog)  Indices=[19]  OutputSizes=1
  Selector3 : Selector  InputPortWidth=21  IndexOptions=Index vector (dialog)  Indices=[12]  OutputSizes=1
  Selector4 : Selector  InputPortWidth=21  IndexOptions=Index vector (dialog)  Indices=[17]  OutputSizes=1
  Selector5 : Selector  InputPortWidth=21  IndexOptions=Index vector (dialog)  Indices=[18]  OutputSizes=1
  Selector6 : Selector  InputPortWidth=21  IndexOptions=Index vector (dialog)  Indices=[16]  OutputSizes=1
  Selector7 : Selector  InputPortWidth=21  IndexOptions=Index vector (dialog)  Indices=[11]  OutputSizes=1
  Selector8 : Selector  InputPortWidth=21  IndexOptions=Index vector (dialog)  Indices=[10]  OutputSizes=1
  Selector9 : Selector  InputPortWidth=21  IndexOptions=Index vector (dialog)  Indices=[4]  OutputSizes=1
  Traj2State2 : Subsystem
  state : Outport
  wires:
  Mux9/1 -> ApplyRotation2/2, ApplyRotation1/2, ApplyRotation/2
  Selector20/1 -> Mux9/3
  Selector19/1 -> Mux9/2
  Selector21/1 -> Mux9/1
  Selector5/1 -> Mux8/3
  Selector4/1 -> Mux8/2
  Selector6/1 -> Mux8/1
  Mux8/1 -> Mux/6
  Mux6/1 -> ApplyRotation2/1
  Mux7/1 -> Mux/4
  ApplyRotation2/1 -> Mux/5
  Selector3/1 -> Mux7/3
  Selector7/1 -> Mux7/2
  Selector8/1 -> Mux7/1
  Mux4/1 -> Mux/2
  Mux5/1 -> ApplyRotation1/1
  ApplyRotation1/1 -> Mux/3
  Mux2/1 -> ApplyRotation/1
  ApplyRotation/1 -> Mux/1
  Selector2/1 -> Mux4/3
  Selector1/1 -> Mux4/2
  Selector9/1 -> Mux4/1
  Selector17/1 -> Mux6/3
  Selector16/1 -> Mux6/2
  Selector18/1 -> Mux6/1
  Selector14/1 -> Mux5/3
  Selector13/1 -> Mux5/2
  Selector15/1 -> Mux5/1
  Selector11/1 -> Mux2/3
  Selector10/1 -> Mux2/2
  Selector12/1 -> Mux2/1
  Mux3/1 -> Selector8/1, Selector7/1, Selector3/1, Selector18/1, Selector16/1, Selector17/1, Selector6/1, Selector20/1, Selector19/1, Selector21/1, Selector5/1, Selector4/1, Selector14/1, Selector13/1, Selector15/1, Selector2/1, Selector1/1, Selector9/1, Selector12/1, Selector10/1, Selector11/1
  Mux1/1 -> Add2/2
  Constant/1 -> Mux1/2
  Add2/1 -> Traj2State2/1(traj)
  Selector/1 -> Mux3/2
  Traj Org/1 -> Mux3/1
  Offset/1 -> Mux1/1, Selector/1
  Mux/1 -> Add2/1
  Traj2State2/1(state) -> state/1

== system Demo_DSRC_BSM_Message_cs/Citroen_C3_1/Trajectories/Trajectory_3 ==
  From Workspace : FromWorkspace  VariableName=trajectory  SampleTime=TimeStep  OutputAfterFinalValue=Holding final value
  From Workspace1 : FromWorkspace  VariableName=trajectory  SampleTime=TimeStep  OutputAfterFinalValue=Setting to zero
  Mux : Mux  Inputs=2
  Selector1 : Selector  InputPortWidth=24  IndexOptions=Index vector (dialog)  Indices=[7:18]  OutputSizes=1
  Selector9 : Selector  InputPortWidth=24  IndexOptions=Index vector (dialog)  Indices=[1:6]  OutputSizes=1
  trajectory : Outport
  wires:
  Selector1/1 -> Mux/2
  Selector9/1 -> Mux/1
  Mux/1 -> trajectory/1
  From Workspace1/1 -> Selector1/1
  From Workspace/1 -> Selector9/1

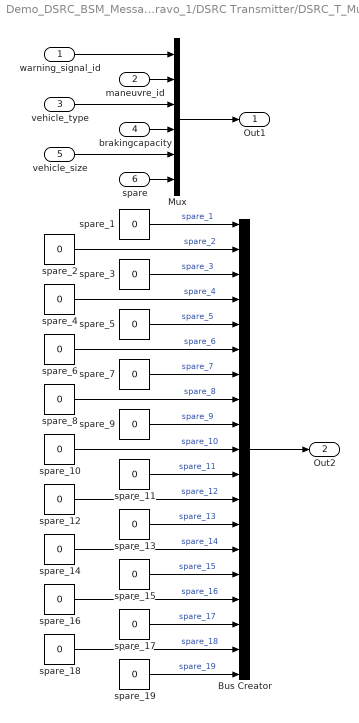
== system Demo_DSRC_BSM_Message_cs/Fiat_Bravo_1/DSRC Transmitter/DSRC_T_Mux ==
  warning_signal_id : Inport
  maneuvre_id : Inport  Port=2
  vehicle_type : Inport  Port=3
  brakingcapacity : Inport  Port=4
  vehicle_size : Inport  Port=5
  spare : Inport  Port=6
  Bus Creator : BusCreator  Inputs=19
  Mux : Mux  Inputs=6
  spare_{1..19} (19 alike) : Constant  Value=0
  Out1 : Outport
  Out2 : Outport  Port=2
  wires:
  spare_3/1 -> Bus Creator/3  "spare_3"
  spare_2/1 -> Bus Creator/2  "spare_2"
  spare_1/1 -> Bus Creator/1  "spare_1"
  spare_4/1 -> Bus Creator/4  "spare_4"
  spare/1 -> Mux/6
  Bus Creator/1 -> Out2/1
  Mux/1 -> Out1/1
  vehicle_size/1 -> Mux/5
  brakingcapacity/1 -> Mux/4
  vehicle_type/1 -> Mux/3
  maneuvre_id/1 -> Mux/2
  warning_signal_id/1 -> Mux/1
  spare_5/1 -> Bus Creator/5  "spare_5"
  spare_6/1 -> Bus Creator/6  "spare_6"
  spare_7/1 -> Bus Creator/7  "spare_7"
  spare_8/1 -> Bus Creator/8  "spare_8"
  spare_9/1 -> Bus Creator/9  "spare_9"
  spare_10/1 -> Bus Creator/10  "spare_10"
  spare_11/1 -> Bus Creator/11  "spare_11"
  spare_12/1 -> Bus Creator/12  "spare_12"
  spare_13/1 -> Bus Creator/13  "spare_13"
  spare_14/1 -> Bus Creator/14  "spare_14"
  spare_15/1 -> Bus Creator/15  "spare_15"
  spare_16/1 -> Bus Creator/16  "spare_16"
  spare_17/1 -> Bus Creator/17  "spare_17"
  spare_18/1 -> Bus Creator/18  "spare_18"
  spare_19/1 -> Bus Creator/19  "spare_19"

== system Demo_DSRC_BSM_Message_cs/Fiat_Bravo_1/SELF_Demux/compas converter ==
  rotz [rad] : Inport
  cart2compas : Subsystem
  rad2deg : Gain  Gain=180/pi
  heading [deg] : Outport
  wires:
  cart2compas/1(heading [deg]) -> heading [deg]/1
  rotz [rad]/1 -> rad2deg/1
  rad2deg/1 -> cart2compas/1(Angle [deg])

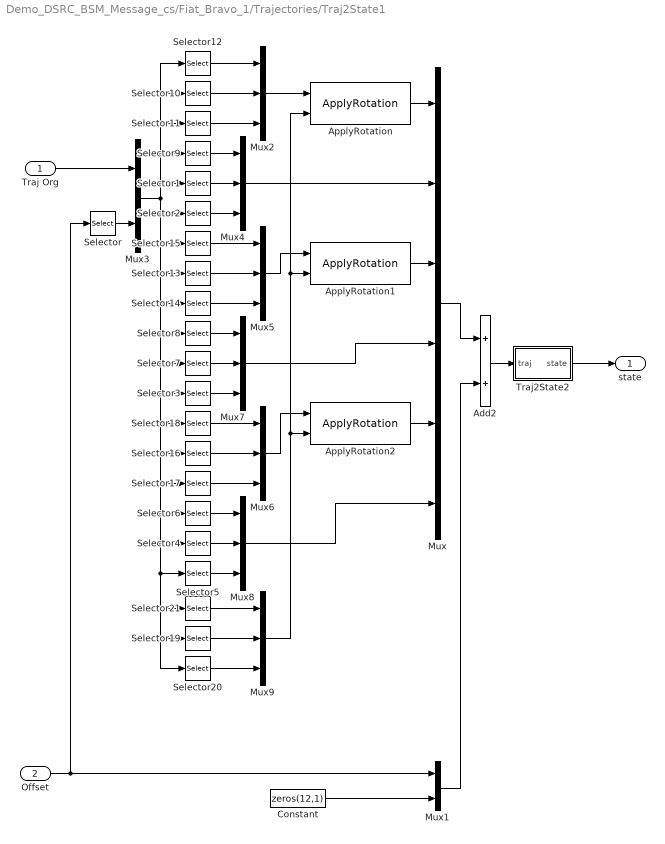
== system Demo_DSRC_BSM_Message_cs/Fiat_Bravo_1/Trajectories/Traj2State1 ==
  Traj Org : Inport
  Offset : Inport  Port=2
  Add2 : Sum
  ApplyRotation : PreScanSimulinkLibrary/ApplyRotation
  ApplyRotation1 : PreScanSimulinkLibrary/ApplyRotation
  ApplyRotation2 : PreScanSimulinkLibrary/ApplyRotation
  Constant : Constant  Value=zeros(12,1)
  Mux : Mux  Inputs=6
  Mux1 : Mux  Inputs=2
  Mux{2,4..9} (7 alike) : Mux  Inputs=3
  Mux3 : Mux  Inputs=2
  Selector : Selector  InputPortWidth=6  IndexOptions=Index vector (dialog)  Indices=[4 5 6]  OutputSizes=1
  Selector1 : Selector  InputPortWidth=21  IndexOptions=Index vector (dialog)  Indices=[5]  OutputSizes=1
  Selector10 : Selector  InputPortWidth=21  IndexOptions=Index vector (dialog)  Indices=[2]  OutputSizes=1
  Selector11 : Selector  InputPortWidth=21  IndexOptions=Index vector (dialog)  Indices=[3]  OutputSizes=1
  Selector12 : Selector  InputPortWidth=21  IndexOptions=Index vector (dialog)  Indices=[1]  OutputSizes=1
  Selector13 : Selector  InputPortWidth=21  IndexOptions=Index vector (dialog)  Indices=[8]  OutputSizes=1
  Selector14 : Selector  InputPortWidth=21  IndexOptions=Index vector (dialog)  Indices=[9]  OutputSizes=1
  Selector15 : Selector  InputPortWidth=21  IndexOptions=Index vector (dialog)  Indices=[7]  OutputSizes=1
  Selector16 : Selector  InputPortWidth=21  IndexOptions=Index vector (dialog)  Indices=[14]  OutputSizes=1
  Selector17 : Selector  InputPortWidth=21  IndexOptions=Index vector (dialog)  Indices=[15]  OutputSizes=1
  Selector18 : Selector  InputPortWidth=21  IndexOptions=Index vector (dialog)  Indices=[13]  OutputSizes=1
  Selector19 : Selector  InputPortWidth=21  IndexOptions=Index vector (dialog)  Indices=[20]  OutputSizes=1
  Selector2 : Selector  InputPortWidth=21  IndexOptions=Index vector (dialog)  Indices=[6]  OutputSizes=1
  Selector20 : Selector  InputPortWidth=21  IndexOptions=Index vector (dialog)  Indices=[21]  OutputSizes=1
  Selector21 : Selector  InputPortWidth=21  IndexOptions=Index vector (dialog)  Indices=[19]  OutputSizes=1
  Selector3 : Selector  InputPortWidth=21  IndexOptions=Index vector (dialog)  Indices=[12]  OutputSizes=1
  Selector4 : Selector  InputPortWidth=21  IndexOptions=Index vector (dialog)  Indices=[17]  OutputSizes=1
  Selector5 : Selector  InputPortWidth=21  IndexOptions=Index vector (dialog)  Indices=[18]  OutputSizes=1
  Selector6 : Selector  InputPortWidth=21  IndexOptions=Index vector (dialog)  Indices=[16]  OutputSizes=1
  Selector7 : Selector  InputPortWidth=21  IndexOptions=Index vector (dialog)  Indices=[11]  OutputSizes=1
  Selector8 : Selector  InputPortWidth=21  IndexOptions=Index vector (dialog)  Indices=[10]  OutputSizes=1
  Selector9 : Selector  InputPortWidth=21  IndexOptions=Index vector (dialog)  Indices=[4]  OutputSizes=1
  Traj2State2 : Subsystem
  state : Outport
  wires:
  Mux9/1 -> ApplyRotation2/2, ApplyRotation1/2, ApplyRotation/2
  Selector20/1 -> Mux9/3
  Selector19/1 -> Mux9/2
  Selector21/1 -> Mux9/1
  Selector5/1 -> Mux8/3
  Selector4/1 -> Mux8/2
  Selector6/1 -> Mux8/1
  Mux8/1 -> Mux/6
  Mux6/1 -> ApplyRotation2/1
  Mux7/1 -> Mux/4
  ApplyRotation2/1 -> Mux/5
  Selector3/1 -> Mux7/3
  Selector7/1 -> Mux7/2
  Selector8/1 -> Mux7/1
  Mux4/1 -> Mux/2
  Mux5/1 -> ApplyRotation1/1
  ApplyRotation1/1 -> Mux/3
  Mux2/1 -> ApplyRotation/1
  ApplyRotation/1 -> Mux/1
  Selector2/1 -> Mux4/3
  Selector1/1 -> Mux4/2
  Selector9/1 -> Mux4/1
  Selector17/1 -> Mux6/3
  Selector16/1 -> Mux6/2
  Selector18/1 -> Mux6/1
  Selector14/1 -> Mux5/3
  Selector13/1 -> Mux5/2
  Selector15/1 -> Mux5/1
  Selector11/1 -> Mux2/3
  Selector10/1 -> Mux2/2
  Selector12/1 -> Mux2/1
  Mux3/1 -> Selector8/1, Selector7/1, Selector3/1, Selector18/1, Selector16/1, Selector17/1, Selector6/1, Selector20/1, Selector19/1, Selector21/1, Selector5/1, Selector4/1, Selector14/1, Selector13/1, Selector15/1, Selector2/1, Selector1/1, Selector9/1, Selector12/1, Selector10/1, Selector11/1
  Mux1/1 -> Add2/2
  Constant/1 -> Mux1/2
  Add2/1 -> Traj2State2/1(traj)
  Selector/1 -> Mux3/2
  Traj Org/1 -> Mux3/1
  Offset/1 -> Mux1/1, Selector/1
  Mux/1 -> Add2/1
  Traj2State2/1(state) -> state/1

== system Demo_DSRC_BSM_Message_cs/Fiat_Bravo_1/Trajectories/Trajectory_2 ==
  From Workspace : FromWorkspace  VariableName=trajectory  SampleTime=TimeStep  OutputAfterFinalValue=Holding final value
  From Workspace1 : FromWorkspace  VariableName=trajectory  SampleTime=TimeStep  OutputAfterFinalValue=Setting to zero
  Mux : Mux  Inputs=2
  Selector1 : Selector  InputPortWidth=24  IndexOptions=Index vector (dialog)  Indices=[7:18]  OutputSizes=1
  Selector9 : Selector  InputPortWidth=24  IndexOptions=Index vector (dialog)  Indices=[1:6]  OutputSizes=1
  trajectory : Outport
  wires:
  Selector1/1 -> Mux/2
  Selector9/1 -> Mux/1
  Mux/1 -> trajectory/1
  From Workspace1/1 -> Selector1/1
  From Workspace/1 -> Selector9/1

== system Demo_DSRC_BSM_Message_cs/BMW_Z3_1/DSRC Receiver/DSRC_Rx_Demux/Reorder ==
  In : Inport
  Selector1 : Selector  InputPortWidth=InputPortWidth  IndexOptions=Index vector (dialog)  Indices=Elements  OutputSizes=1
  Out : Outport
  wires:
  In/1 -> Selector1/1
  Selector1/1 -> Out/1

== system Demo_DSRC_BSM_Message_cs/BMW_Z3_1/DSRC Receiver/DSRC_Rx_Demux/compas converter ==
  rotz [rad] : Inport
  cart2compas : Subsystem
  rad2deg : Gain  Gain=180/pi
  heading [deg] : Outport
  wires:
  cart2compas/1(heading [deg]) -> heading [deg]/1
  rotz [rad]/1 -> rad2deg/1
  rad2deg/1 -> cart2compas/1(Angle [deg])

== system Demo_DSRC_BSM_Message_cs/BMW_Z3_1/SELF_Demux/compas converter/cart2compas ==
  Angle [deg] : Inport
  Constant : Constant  Value=90
  Constant1 : Constant  Value=360
  Gain : Gain  Gain=1/360
  Gain1 : Gain  Gain=360
  Gain2 : Gain  Gain=-1
  Rounding Function : Rounding
  Sum : Sum  Inputs=|-+
  Sum1 : Sum  Inputs=-+|
  Sum2 : Sum  Inputs=++|
  heading [deg] : Outport
  wires:
  Sum2/1 -> heading [deg]/1
  Constant1/1 -> Sum2/1
  Gain2/1 -> Sum2/2
  Constant/1 -> Sum1/1
  Sum1/1 -> Sum/2, Gain/1
  Sum/1 -> Gain2/1
  Angle [deg]/1 -> Sum1/2
  Gain1/1 -> Sum/1
  Rounding Function/1 -> Gain1/1
  Gain/1 -> Rounding Function/1

== system Demo_DSRC_BSM_Message_cs/BMW_Z3_1/Trajectories/Traj2State1/Traj2State2 ==
  traj : Inport
  MuxState : Subsystem
  Traj2MuxState_Ext : Subsystem
  state : Outport
  wires:
  Traj2MuxState_Ext/9(Y [rad]) -> MuxState/9(Y [rad])
  Traj2MuxState_Ext/8(P [rad]) -> MuxState/8(P [rad])
  Traj2MuxState_Ext/7(R [rad]) -> MuxState/7(R [rad])
  Traj2MuxState_Ext/6(dz [m/s]) -> MuxState/6(dz [m/s])
  Traj2MuxState_Ext/5(dy [m/s]) -> MuxState/5(dy [m/s])
  Traj2MuxState_Ext/4(dx [m/s]) -> MuxState/4(dx [m/s])
  Traj2MuxState_Ext/3(z [m]) -> MuxState/3(z [m])
  Traj2MuxState_Ext/2(y [m]) -> MuxState/2(y [m])
  Traj2MuxState_Ext/1(x [m]) -> MuxState/1(x [m])
  MuxState/1(state) -> state/1
  traj/1 -> Traj2MuxState_Ext/1(Traj)

== system Demo_DSRC_BSM_Message_cs/Citroen_C3_1/SELF_Demux/compas converter/cart2compas ==
  Angle [deg] : Inport
  Constant : Constant  Value=90
  Constant1 : Constant  Value=360
  Gain : Gain  Gain=1/360
  Gain1 : Gain  Gain=360
  Gain2 : Gain  Gain=-1
  Rounding Function : Rounding
  Sum : Sum  Inputs=|-+
  Sum1 : Sum  Inputs=-+|
  Sum2 : Sum  Inputs=++|
  heading [deg] : Outport
  wires:
  Sum2/1 -> heading [deg]/1
  Constant1/1 -> Sum2/1
  Gain2/1 -> Sum2/2
  Constant/1 -> Sum1/1
  Sum1/1 -> Sum/2, Gain/1
  Sum/1 -> Gain2/1
  Angle [deg]/1 -> Sum1/2
  Gain1/1 -> Sum/1
  Rounding Function/1 -> Gain1/1
  Gain/1 -> Rounding Function/1

== system Demo_DSRC_BSM_Message_cs/Citroen_C3_1/Trajectories/Traj2State1/Traj2State2 ==
  traj : Inport
  MuxState : Subsystem
  Traj2MuxState_Ext : Subsystem
  state : Outport
  wires:
  Traj2MuxState_Ext/9(Y [rad]) -> MuxState/9(Y [rad])
  Traj2MuxState_Ext/8(P [rad]) -> MuxState/8(P [rad])
  Traj2MuxState_Ext/7(R [rad]) -> MuxState/7(R [rad])
  Traj2MuxState_Ext/6(dz [m/s]) -> MuxState/6(dz [m/s])
  Traj2MuxState_Ext/5(dy [m/s]) -> MuxState/5(dy [m/s])
  Traj2MuxState_Ext/4(dx [m/s]) -> MuxState/4(dx [m/s])
  Traj2MuxState_Ext/3(z [m]) -> MuxState/3(z [m])
  Traj2MuxState_Ext/2(y [m]) -> MuxState/2(y [m])
  Traj2MuxState_Ext/1(x [m]) -> MuxState/1(x [m])
  MuxState/1(state) -> state/1
  traj/1 -> Traj2MuxState_Ext/1(Traj)

== system Demo_DSRC_BSM_Message_cs/Fiat_Bravo_1/SELF_Demux/compas converter/cart2compas ==
  Angle [deg] : Inport
  Constant : Constant  Value=90
  Constant1 : Constant  Value=360
  Gain : Gain  Gain=1/360
  Gain1 : Gain  Gain=360
  Gain2 : Gain  Gain=-1
  Rounding Function : Rounding
  Sum : Sum  Inputs=|-+
  Sum1 : Sum  Inputs=-+|
  Sum2 : Sum  Inputs=++|
  heading [deg] : Outport
  wires:
  Sum2/1 -> heading [deg]/1
  Constant1/1 -> Sum2/1
  Gain2/1 -> Sum2/2
  Constant/1 -> Sum1/1
  Sum1/1 -> Sum/2, Gain/1
  Sum/1 -> Gain2/1
  Angle [deg]/1 -> Sum1/2
  Gain1/1 -> Sum/1
  Rounding Function/1 -> Gain1/1
  Gain/1 -> Rounding Function/1

== system Demo_DSRC_BSM_Message_cs/Fiat_Bravo_1/Trajectories/Traj2State1/Traj2State2 ==
  traj : Inport
  MuxState : Subsystem
  Traj2MuxState_Ext : Subsystem
  state : Outport
  wires:
  Traj2MuxState_Ext/9(Y [rad]) -> MuxState/9(Y [rad])
  Traj2MuxState_Ext/8(P [rad]) -> MuxState/8(P [rad])
  Traj2MuxState_Ext/7(R [rad]) -> MuxState/7(R [rad])
  Traj2MuxState_Ext/6(dz [m/s]) -> MuxState/6(dz [m/s])
  Traj2MuxState_Ext/5(dy [m/s]) -> MuxState/5(dy [m/s])
  Traj2MuxState_Ext/4(dx [m/s]) -> MuxState/4(dx [m/s])
  Traj2MuxState_Ext/3(z [m]) -> MuxState/3(z [m])
  Traj2MuxState_Ext/2(y [m]) -> MuxState/2(y [m])
  Traj2MuxState_Ext/1(x [m]) -> MuxState/1(x [m])
  MuxState/1(state) -> state/1
  traj/1 -> Traj2MuxState_Ext/1(Traj)

== system Demo_DSRC_BSM_Message_cs/BMW_Z3_1/DSRC Receiver/DSRC_Rx_Demux/compas converter/cart2compas ==
  Angle [deg] : Inport
  Constant : Constant  Value=90
  Constant1 : Constant  Value=360
  Gain : Gain  Gain=1/360
  Gain1 : Gain  Gain=360
  Gain2 : Gain  Gain=-1
  Rounding Function : Rounding
  Sum : Sum  Inputs=|-+
  Sum1 : Sum  Inputs=-+|
  Sum2 : Sum  Inputs=++|
  heading [deg] : Outport
  wires:
  Sum2/1 -> heading [deg]/1
  Constant1/1 -> Sum2/1
  Gain2/1 -> Sum2/2
  Constant/1 -> Sum1/1
  Sum1/1 -> Sum/2, Gain/1
  Sum/1 -> Gain2/1
  Angle [deg]/1 -> Sum1/2
  Gain1/1 -> Sum/1
  Rounding Function/1 -> Gain1/1
  Gain/1 -> Rounding Function/1

== system Demo_DSRC_BSM_Message_cs/BMW_Z3_1/Trajectories/Traj2State1/Traj2State2/MuxState ==
  x [m] : Inport
  y [m] : Inport  Port=2
  z [m] : Inport  Port=3
  dx [m/s] : Inport  Port=4
  dy [m/s] : Inport  Port=5
  dz [m/s] : Inport  Port=6
  R [rad] : Inport  Port=7
  P [rad] : Inport  Port=8
  Y [rad] : Inport  Port=9
  Mux : Mux  Inputs=9
  state : Outport
  wires:
  z [m]/1 -> Mux/3
  y [m]/1 -> Mux/2
  x [m]/1 -> Mux/1
  Y [rad]/1 -> Mux/9
  P [rad]/1 -> Mux/8
  R [rad]/1 -> Mux/7
  dz [m/s]/1 -> Mux/6
  dy [m/s]/1 -> Mux/5
  dx [m/s]/1 -> Mux/4
  Mux/1 -> state/1
